simulink model "prob_1b"  (R2020a)
settings: Solver=VariableStepAuto  StartTime=0.0  StopTime=10  RelTol=1e-3
values from neighbouring files (symbols this model uses):
  a0 = J/swp^2    (= 1183.43195266)    [params.m]
  a1 = 2*sdr*J/swp + Kd/swz^2    (= 1706.15384615)    [params.m]
  a2 = J + 2*sdr*Kd/swz + Kp/swz^2    (= 3006.8)    [params.m]
  a3 = Kd + 2*sdr*Kp/swz    (= 1704)    [params.m]
  a4 = Kp    (= 1000)    [params.m]
  b0 = Kd/swz^2    (= 1700)    [params.m]
  b1 = Kp/swz^2 + 2*sdr*Kd/swz    (= 1006.8)    [params.m]
  b2 = 2*sdr*Kp/swz + Kd    (= 1704)    [params.m]
  b3 = Kp    (= 1000)    [params.m]
libraries: slctrlblks x1
settings Model: Creator=VTOL_HYD  LastModifiedBy=VTOL_HYD

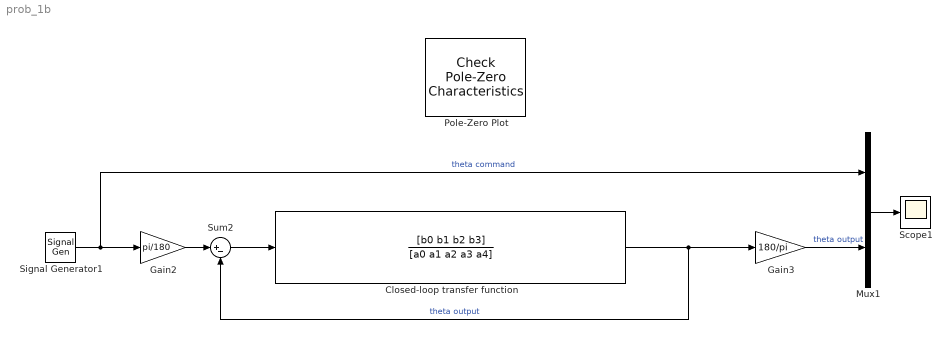
== system prob_1b ==
  Closed-loop transfer function : TransferFcn  Numerator=[b0 b1 b2 b3]  Denominator=[a0 a1 a2 a3 a4]
  Gain2 : Gain  Gain=pi/180
  Gain3 : Gain  Gain=180/pi
  Mux1 : Mux  Inputs=2
  Pole-Zero Plot : slctrlblks/Model Verification/Check Pole-Zero Characteristics  InstantiateOnLoad=on  SaveOperatingPoints=on  LinearizationIOs={'/Sum2', 1, 'in', 'on', '';'/Closed-loop transfer function', 1, 'out', 'on', ''}  LinearizeAt=SnapshotTimes  SnapshotTimes=[0]  TriggerType=rising  SampleTime=auto  RateConversionMethod=zoh  PreWarpFreq=10  UseExactDelayModel=off  UseFullBlockNameLabels=off  UseBusSignalLabels=off  enabled=on  stopWhenAssertionFail=off  export=off  ViewDlgPos=[44 38 958 954]  LaunchViewOnOpen=off  OpenViewOnLoad=off  FrequencyUnits=rad/s  MagnitudeUnits=dB  PhaseUnits=deg  TimeUnits=seconds  EnableSettlingTime=off  SettlingTime=[]  EnablePercentOvershoot=off  PercentOvershoot=[]  EnableDampingRatio=off  DampingRatio=[]  EnableNaturalFrequency=off  NaturalFrequencyBound=>=  NaturalFrequency=[]
      settings: SourceProductBaseCode=SD  SaveToWorkspace=on  SaveName=sys
  Scope1 : Scope
  Signal Generator1 : SignalGenerator  WaveForm=square  Amplitude=30  Units=rad/sec
  Sum2 : Sum  Inputs=|+-
  wires:
  Sum2/1 -> Closed-loop transfer function/1
  Signal Generator1/1 -> Mux1/1, Gain2/1  "theta command"
  Gain2/1 -> Sum2/1
  Gain3/1 -> Mux1/2  "theta output"
  Mux1/1 -> Scope1/1
  Closed-loop transfer function/1 -> Sum2/2, Gain3/1  "theta output"
